simulink model "sim_pil_top_BLDC_Commutation_s32k1xx"  (Simulink 9.0)
settings: Solver=FixedStepDiscrete  StartTime=0.0  StopTime=1.2  FixedStep=0.1  RelTol=1e-3  EnableMultiTasking=on
InitFcn:
  | mbd_s32k_consistency_checks(bdroot(gcs));
libraries: simulink x1
Description:
  | This model demonstrates the PIL concept.
  | The Hall based commutation and PWM control is executed on the S32K144 uP
  | and the results are upleaded via UART into Simulink where it can be compared
  | against the results obtained with sim_sil_top_BLDC_Commutation_s32k14 model
  | 
  | Inputs:
  | - Rotation DIRECTION [CW(1) or CCW(-1)] can be set to 1(clockwise) or -1(counter clockwise).
  | - PWM duty cycle [PWM_Duty_Cycle] can be set to any value between 0-1.
  | 
  | Outputs:
  | Based on DIRECTION the comuttation sequence for each phase is updated.
  | - [PWM_A_HS_out] represents the PWM command for High Switch on Phase A
  | - [PWM_A_LS_out] represents the PWM command for Low Switch on Phase A
  | - [PWM_B_HS_out] represents the PWM command for High Switch on Phase B
  | - [PWM_B_LS_out] represents the PWM command for Low Switch on Phase B
  | - [PWM_C_HS_out] represents the PWM command for High Switch on Phase C
  | - [PWM_C_LS_out] represents the PWM command for Low Switch on Phase C
  | 
  | The output(0...1) of the PIL Model should be identical compared to results of SIL Model.
settings Model: Creator=NXP MBDT Team  LastModifiedBy=nxf35172
settings DataIOCC: ExternalInput=off  InitialState=off  LimitDataPoints=on  SaveOutput=off  SignalLogging=off  SaveTime=off
settings OptimizationCC: DefaultParameterBehavior=Inlined  PassReuseOutputArgsAs=Individual arguments  LifeSpan=auto
settings DebuggingCC: UnderspecifiedInitializationDetection=Simplified  MergeDetectMultiDrivingBlocksExec=error  SolverPrmCheckMsg=warning  InheritedTsInSrcMsg=none  SingleTaskRateTransMsg=error  ParameterTunabilityLossMsg=error  UnconnectedInputMsg=error  UnconnectedOutputMsg=error  UnconnectedLineMsg=error  AllowSymbolicDim=off  UnknownTsInhSupMsg=error
settings HardwareCC: ProdLargestAtomicInteger=Long  ProdLargestAtomicFloat=Double  ProdIntDivRoundTo=Zero  ProdEndianess=LittleEndian  ProdHWDeviceType=ARM Compatible->ARM Cortex
settings SFSimCC: MATLABDynamicMemAlloc=off
settings RTWCC: SystemTargetFile=mbd_s32k.tlc  MakeCommand=mbd_s32k_make_rtw COPY_MDLREF_INCLUDES=0  TemplateMakefile=mbd_s32k.tmf  Description=Model Based Design Toolbox S32K1xx Code Generation Target  GenerateReport=on  IncludeHyperlinkInReport=on  LaunchReport=on  CreateSILPILBlock=PIL  GenerateTraceInfo=on  GenerateTraceReport=on  GenerateTraceReportSl=on  GenerateTraceReportSf=on  GenerateTraceReportEml=on
settings CodeAppCC: ForceParamTrailComments=on  IgnoreCustomStorageClasses=off  MaxIdLength=63  OperatorAnnotations=on  SimulinkDataObjDesc=on  SFDataObjDesc=on  InsertBlockDesc=on  StateflowObjectComments=off
settings STFCustomTargetCC: MultiwordLength=256  GenerateSampleERTMain=on  CombineOutputUpdateFcns=on  ERTCustomFileBanners=on  SupportContinuousTime=off  SupportNonInlinedSFcns=off  RemoveResetFunc=on  MATLABClassNameForMDSCustomization=Simulink.SoftwareTarget.ERTCustomization  GRTInterface=off  SystemTargetFile=mbd_s32k.tlc
settings ERTTargetCC: GenerateSampleERTMain=on  ParMdlRefBuildCompliant=off  CompOptLevelCompliant=off  ConcurrentExecutionCompliant=off  ModelStepFunctionPrototypeControlCompliant=off  CPPClassGenCompliant=off  UseToolchainInfoCompliant=off  InlinedParameterPlacement=NonHierarchical  ERTSrcFileBannerTemplate=mbd_ert_code_template.cgt  ERTHdrFileBannerTemplate=mbd_ert_code_template.cgt  ERTDataSrcFileTemplate=mbd_ert_code_template.cgt  ERTDataHdrFileTemplate=mbd_ert_code_template.cgt  ERTCustomFileTemplate=example_file_process.tlc

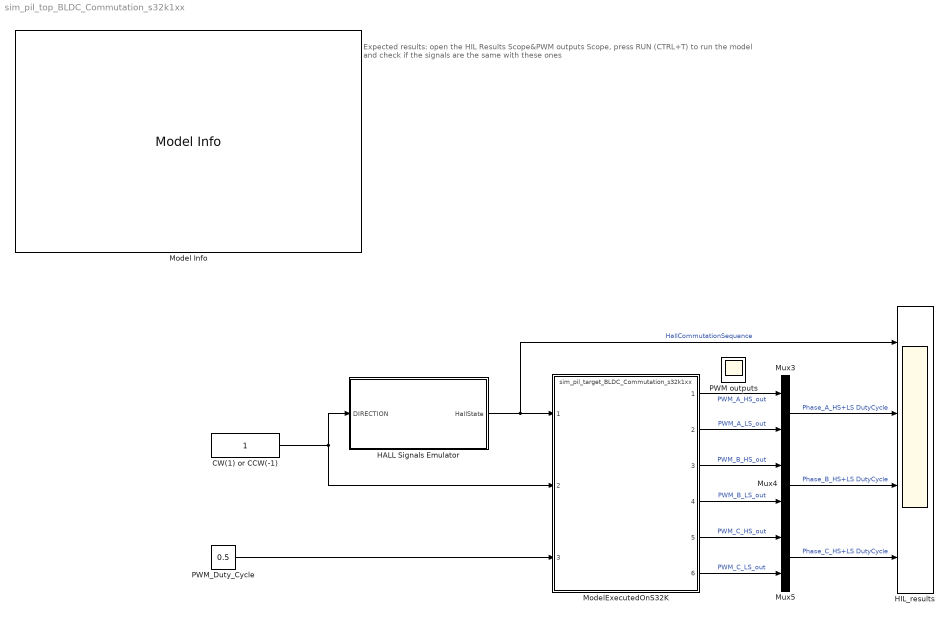
== system sim_pil_top_BLDC_Commutation_s32k1xx ==
  note: Expected results: open the HIL Results Scope&PWM outputs Scope, press RUN (CTRL+T) to run the model and check if the signals are the same with these ones
  CW(1) or CCW(-1) : Constant  OutMin=-1  OutMax=1  OutDataTypeStr=single
  HALL Signals Emulator : Subsystem
  HIL_results : Scope  NumInputPorts=4
  Model Info : simulink/Model-Wide Utilities/Model Info  Frame=off  DisplayStringWithTags=|  HorizontalTextAlignment=Left  LeftAlignmentValue=0.02
      | Model Name: %<ModelName>
      | 
      | Description: %<Description>
  ModelExecutedOnS32K : ModelReference  ModelNameDialog=sim_pil_target_BLDC_Commutation_s32k1xx.mdl  SimulationMode=Processor-in-the-loop (PIL)  ModelReferenceVersion=1.104
  Mux3 : Mux  Inputs=2
  Mux4 : Mux  Inputs=2
  Mux5 : Mux  Inputs=2
  PWM outputs : Scope
      settings: Floating=on
  PWM_Duty_Cycle : Constant  Value=0.5  OutMin=0  OutMax=100  OutDataTypeStr=single
  wires:
  CW(1) or CCW(-1)/1 -> ModelExecutedOnS32K/2, HALL Signals Emulator/1(DIRECTION)
  PWM_Duty_Cycle/1 -> ModelExecutedOnS32K/3
  HALL Signals Emulator/1(HallState) -> HIL_results/1, ModelExecutedOnS32K/1  "HallCommutationSequence"
  Mux3/1 -> HIL_results/2  "Phase_A_HS+LS DutyCycle"
  Mux4/1 -> HIL_results/3  "Phase_B_HS+LS DutyCycle"
  Mux5/1 -> HIL_results/4  "Phase_C_HS+LS DutyCycle"
  ModelExecutedOnS32K/1 -> Mux3/1  "PWM_A_HS_out"
  ModelExecutedOnS32K/2 -> Mux3/2  "PWM_A_LS_out"
  ModelExecutedOnS32K/3 -> Mux4/1  "PWM_B_HS_out"
  ModelExecutedOnS32K/4 -> Mux4/2  "PWM_B_LS_out"
  ModelExecutedOnS32K/5 -> Mux5/1  "PWM_C_HS_out"
  ModelExecutedOnS32K/6 -> Mux5/2  "PWM_C_LS_out"

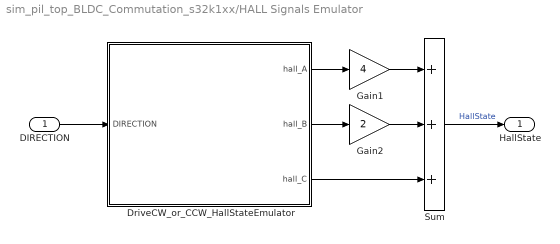
== system sim_pil_top_BLDC_Commutation_s32k1xx/HALL Signals Emulator ==
  DIRECTION : Inport
  DriveCW_or_CCW_HallStateEmulator : Stateflow chart  TreatAsAtomicUnit=on
  Gain1 : Gain  Gain=4  OutDataTypeStr=uint8  ParamDataTypeStr=Inherit: Same as input
  Gain2 : Gain  Gain=2  OutDataTypeStr=uint8  ParamDataTypeStr=Inherit: Same as input
  Sum : Sum  Inputs=+++  AccumDataTypeStr=uint8  OutDataTypeStr=uint8
  HallState : Outport
  wires:
  Sum/1 -> HallState/1  "HallState"
  Gain2/1 -> Sum/2
  DriveCW_or_CCW_HallStateEmulator/2(hall_B) -> Gain2/1
  Gain1/1 -> Sum/1
  DriveCW_or_CCW_HallStateEmulator/3(hall_C) -> Sum/3
  DriveCW_or_CCW_HallStateEmulator/1(hall_A) -> Gain1/1
  DIRECTION/1 -> DriveCW_or_CCW_HallStateEmulator/1(DIRECTION)

== stateflow chart HALL Signals Emulator/DriveCW_or_CCW_HallStateEmulator ==
  state STEP1
    entry:
    hall_A = uint8(1);
    hall_B = uint8(0);
    hall_C = uint8(0);
  state STEP2_CCW
    entry:
    hall_A = uint8(1);
    hall_B = uint8(0);
    hall_C = uint8(1);
  state STEP2_CW
    entry:
    hall_A = uint8(1);
    hall_B = uint8(1);
    hall_C = uint8(0);
  state STEP3_CCW
    entry:
    hall_A = uint8(0);
    hall_B = uint8(0);
    hall_C = uint8(1);
  state STEP3
    entry:
    hall_A = uint8(0);
    hall_B = uint8(1);
    hall_C = uint8(0);
  state STEP4_CCW
    entry:
    hall_A = uint8(0);
    hall_B = uint8(1);
    hall_C = uint8(1);
  state STEP4
    entry:
    hall_A = uint8(0);
    hall_B = uint8(1);
    hall_C = uint8(1);
  state STEP5_CCW
    entry:
    hall_A = uint8(0);
    hall_B = uint8(1);
    hall_C = uint8(0);
  state STEP5
    entry:
    hall_A = uint8(0);
    hall_B = uint8(0);
    hall_C = uint8(1);
  state STEP6_CCW
    entry:
    hall_A = uint8(1);
    hall_B = uint8(1);
    hall_C = uint8(0);
  state STEP6
    entry:
    hall_A = uint8(1);
    hall_B = uint8(0);
    hall_C = uint8(1);
  (default) -> STEP1
  STEP1 -> STEP2_CW [order 1] : [DIRECTION >=0]
  STEP1 -> STEP2_CCW [order 2] : [DIRECTION<0]
  STEP6_CCW -> STEP1
  STEP6 -> STEP1
  STEP2_CW -> STEP3
  STEP2_CCW -> STEP3_CCW
  STEP3_CCW -> STEP4_CCW
  STEP3 -> STEP4
  STEP4_CCW -> STEP5_CCW
  STEP4 -> STEP5
  STEP5_CCW -> STEP6_CCW
  STEP5 -> STEP6
  data: hall_A output uint8; hall_B output uint8; hall_C output uint8; DIRECTION input single
